simulink model "mainmodel"  (R2020a)
settings: Solver=VariableStepAuto  StartTime=0.0  StopTime=10.0  RelTol=1e-3
PreLoadFcn:
  | a1 = 0.5;
  | a2 = 0.25;
  | b2 = 0.4;
settings Model: Creator=Bhanu  LastModifiedBy=Bhanu

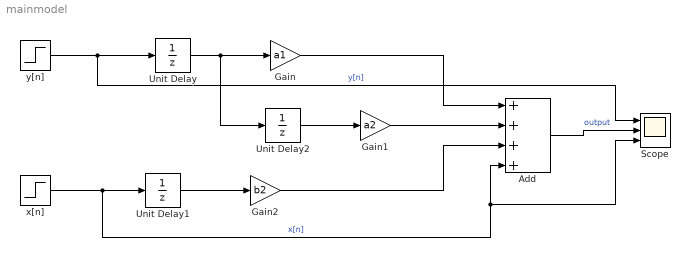
== system mainmodel ==
  Add : Sum  Inputs=++++
  Gain : Gain  Gain=a1
  Gain1 : Gain  Gain=a2
  Gain2 : Gain  Gain=b2
  Scope : Scope  NumInputPorts=3
  Unit Delay : UnitDelay  SampleTime=-1  HasFrameUpgradeWarning=on
  Unit Delay1 : UnitDelay  SampleTime=-1  HasFrameUpgradeWarning=on
  Unit Delay2 : UnitDelay  SampleTime=-1  HasFrameUpgradeWarning=on
  x[n] : Step  SampleTime=0
  y[n] : Step  SampleTime=0
  wires:
  y[n]/1 -> Scope/1, Unit Delay/1  "y[n]"
  x[n]/1 -> Scope/3, Add/4, Unit Delay1/1  "x[n]"
  Unit Delay/1 -> Unit Delay2/1, Gain/1
  Unit Delay2/1 -> Gain1/1
  Unit Delay1/1 -> Gain2/1
  Gain/1 -> Add/1
  Gain1/1 -> Add/2
  Gain2/1 -> Add/3
  Add/1 -> Scope/2  "output"
